simulink model "frame_inspector_test"  (R2020a)
settings: Solver=VariableStepAuto  StartTime=0.0  StopTime=(4096*6)/1e6  RelTol=1e-3
undefined symbols (not defined in the file): frame_size
libraries: hdlsllib x3, dspsrcs4 x2, dspsigops x2
settings Model: Creator=LDM  LastModifiedBy=LDM
settings OptimizationCC: BlockReduction=off  ConditionallyExecuteInputs=off  DefaultParameterBehavior=Inlined
settings DebuggingCC: AlgebraicLoopMsg=error
settings HardwareCC: ProdBitPerPointer=32  ProdBitPerSizeT=32  ProdBitPerPtrDiffT=32  ProdLargestAtomicFloat=None  ProdIntDivRoundTo=Undefined  ProdEndianess=Unspecified  ProdWordSize=32  ProdHWDeviceType=ASIC/FPGA->ASIC/FPGA  TargetBitPerPointer=64  TargetBitPerSizeT=64  TargetBitPerPtrDiffT=64  TargetLongLongMode=on  TargetIntDivRoundTo=Zero  TargetEndianess=LittleEndian  TargetWordSize=64  TargetHWDeviceType=Custom Processor->MATLAB Host Computer  ProdEqTarget=off

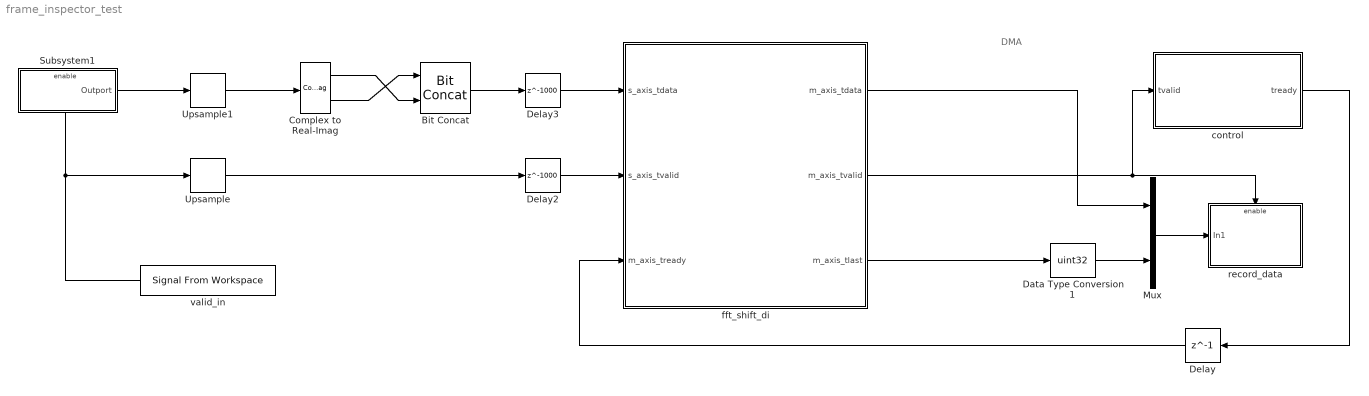
== system frame_inspector_test ==
  note: DMA
  Bit Concat : hdlsllib/Logic and Bit Operations/Bit Concat  numInputs=2
  Complex to Real-Imag : ComplexToRealImag
  Data Type Conversion1 : DataTypeConversion  OutDataTypeStr=uint32
  Delay : Delay  DelayLength=1
  Delay2 : Delay  DelayLength=1000
  Delay3 : Delay  DelayLength=1000
  Mux : Mux  Inputs=2
  Subsystem1 : Subsystem
  Upsample : dspsigops/Upsample  N=12  phase=0  RateOptions=Allow multirate processing  ic=0  mode=Unused parameter value
  Upsample1 : dspsigops/Upsample  N=12  phase=0  RateOptions=Allow multirate processing  ic=0  mode=Unused parameter value
  control : Stateflow chart  TreatAsAtomicUnit=on
  fft_shift_di : Subsystem  TreatAsAtomicUnit=on
  record_data : Subsystem
  valid_in : dspsrcs4/Signal From Workspace  X=[true(1,randi(10)) false(1,randi(10)) true(1,randi(10))]  Ts=1/1e6  nsamps=1  OutputAfterFinalValue=Cyclic repetition  ignoreOrWarnInputAndFrameLengths=off  OutputFrames=off
  wires:
  control/1(tready) -> Delay/1
  Subsystem1/1(Outport) -> Upsample1/1
  valid_in/1 -> Upsample/1, Subsystem1/Enable
  Upsample1/1 -> Complex to Real-Imag/1
  Delay/1 -> fft_shift_di/3(m_axis_tready)
  Mux/1 -> record_data/1(In1)
  fft_shift_di/1(m_axis_tdata) -> Mux/1
  Complex to Real-Imag/1 -> Bit Concat/2
  Complex to Real-Imag/2 -> Bit Concat/1
  Upsample/1 -> Delay2/1
  fft_shift_di/2(m_axis_tvalid) -> control/1(tvalid), record_data/Enable
  fft_shift_di/3(m_axis_tlast) -> Data Type Conversion1/1
  Data Type Conversion1/1 -> Mux/2
  Bit Concat/1 -> Delay3/1
  Delay2/1 -> fft_shift_di/2(s_axis_tvalid)
  Delay3/1 -> fft_shift_di/1(s_axis_tdata)

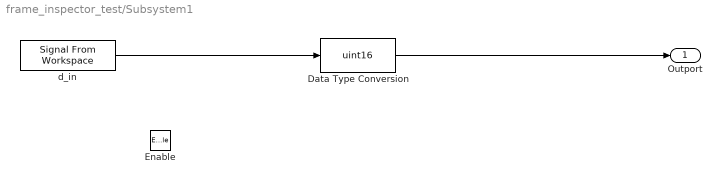
== system frame_inspector_test/Subsystem1 ==
  Enable : EnablePort
  Data Type Conversion : DataTypeConversion  OutDataTypeStr=uint16
  d_in : dspsrcs4/Signal From Workspace  X=1:frame_size  Ts=1/1e6  nsamps=1  OutputAfterFinalValue=Cyclic repetition  ignoreOrWarnInputAndFrameLengths=off  OutputFrames=off
  Outport : Outport
  wires:
  d_in/1 -> Data Type Conversion/1
  Data Type Conversion/1 -> Outport/1

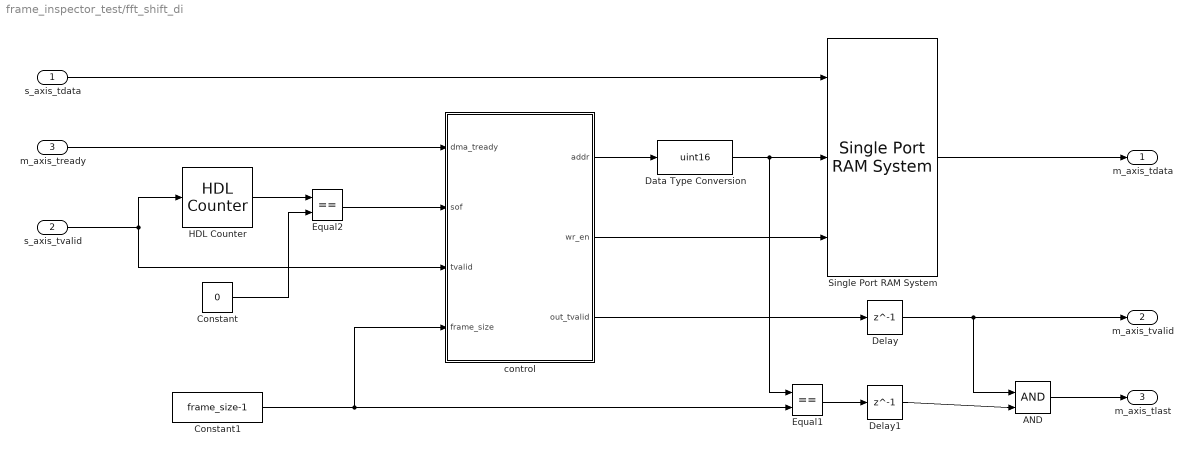
== system frame_inspector_test/fft_shift_di ==
  s_axis_tdata : Inport
  s_axis_tvalid : Inport  Port=2
  m_axis_tready : Inport  Port=3
  AND : Logic  IconShape=distinctive  AllPortsSameDT=off  OutDataTypeStr=boolean
  Constant : Constant  Value=0  OutDataTypeStr=uint16  SampleTime=-1
  Constant1 : Constant  Value=frame_size-1  OutDataTypeStr=uint16  SampleTime=-1
  Data Type Conversion : DataTypeConversion  OutDataTypeStr=uint16
  Delay : Delay  DelayLength=1
  Delay1 : Delay  DelayLength=1
  Equal1 : RelationalOperator  Operator===  OutDataTypeStr=boolean  RndMeth=Simplest
  Equal2 : RelationalOperator  Operator===  OutDataTypeStr=boolean  RndMeth=Simplest
  HDL Counter : hdlsllib/Sources/HDL Counter  CountType=Free running  CountInit=0  CountStep=1  CountMax=63  CountFromType=Initial value  CountFrom=0  CountResetPort=off  CountLoadPort=off  CountEnbPort=on  CountDirPort=off  CountDataType=Unsigned  CountWordLen=log2(frame_size)  CountFracLen=0  CountSampTime=1
  Single Port RAM System : hdlsllib/HDL RAMs/Single Port RAM System  RAMType=Single port  WriteOutputValue=New data  RAMInitialValue=0  SimulateUsing=Code generation
      settings: SourceProductBaseCode=SL
  control : Stateflow chart  TreatAsAtomicUnit=on
  m_axis_tdata : Outport
  m_axis_tvalid : Outport  Port=2
  m_axis_tlast : Outport  Port=3
  wires:
  s_axis_tvalid/1 -> control/3(tvalid), HDL Counter/1
  HDL Counter/1 -> Equal2/1
  Equal2/1 -> control/2(sof)
  Constant/1 -> Equal2/2
  s_axis_tdata/1 -> Single Port RAM System/1
  control/1(addr) -> Data Type Conversion/1
  control/2(wr_en) -> Single Port RAM System/3
  m_axis_tready/1 -> control/1(dma_tready)
  control/3(out_tvalid) -> Delay/1
  Single Port RAM System/1 -> m_axis_tdata/1
  Delay/1 -> m_axis_tvalid/1, AND/1
  Data Type Conversion/1 -> Equal1/1, Single Port RAM System/2
  Constant1/1 -> control/4(frame_size), Equal1/2
  Equal1/1 -> Delay1/1
  Delay1/1 -> AND/2
  AND/1 -> m_axis_tlast/1

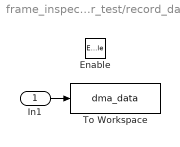
== system frame_inspector_test/record_data ==
  In1 : Inport
  Enable : EnablePort
  To Workspace : ToWorkspace  VariableName=dma_data  SampleTime=-1
      settings: Save2DSignal=2-D array (concatenate along first dimension)
  wires:
  In1/1 -> To Workspace/1

== stateflow chart frame_inspector_test/control ==
  state init
    % variables
    count = 0;
    d_count = 0;
  state start_frame
    %variables
    if tvalid == true
    d_count = d_count + 1
    end
    %outputs
    tready = true
  state wait
    % variables
    count = count + 1;
    %outputs
    tready = false
  state pause
    % variables
    count = count + 1;
    %outputs
    tready = false
  state end_frame
    %variables
    if tvalid == true
    d_count = d_count + 1
    end
    %outputs
    tready = true
  (default) -> init
  init -> wait
  wait -> start_frame : [count > randi(100)]{count = 0}
  end_frame -> wait : [d_count == frame_size]{d_count = 0}
  start_frame -> pause : [d_count == 3]
  pause -> end_frame : [count > randi(100)]{count = 0}
  data: tready output boolean; d_count local; count local; tvalid input; frame_size constant double =frame_size

== stateflow chart frame_inspector_test/fft_shift_di/control ==
  settings: executeAtInitialization=1
  state init
    % variables
    read_flag = false;
    % outputs
    addr=-1;
    wr_en = false;
    out_tvalid = false
  state write
    % variables
    if dma_tready
    read_flag = true;
    end
    % outputs
    addr=addr+1;
    wr_en = true;
    out_tvalid = false
  state idle
    % variables
    if dma_tready
    read_flag = true;
    end
    % outputs
    addr=addr;
    wr_en = false;
    out_tvalid = false
  state wait_update
    % variables
    % outputs
    addr=addr;
    wr_en = false;
    out_tvalid = false
  state wait
    % variables
    if dma_tready
    read_flag = true;
    end
    % outputs
    addr=addr;
    wr_en = false;
    out_tvalid = false
  state read
    % variables
    % outputs
    addr=addr+1;
    wr_en = false;
    out_tvalid = true
  state read_idle
    % variables
    % outputs
    addr=addr;
    wr_en = false;
    out_tvalid = false
  (default) -> init
  init -> write : [sof && tvalid]
  wait_update -> write : [sof && tvalid]
  wait -> write [order 1] : [sof && tvalid]
  write -> idle [order 3] : [~tvalid]
  idle -> write : [tvalid]
  write -> wait [order 2] : [addr==frame_size]
  write -> read [order 1] : [read_flag && addr==frame_size]{read_flag=false;addr=-1}
  read -> wait_update [order 1] : [addr==frame_size]{addr=-1}
  wait -> read [order 2] : [read_flag]{read_flag=false; addr=-1}
  read_idle -> read : [dma_tready]
  read -> read_idle [order 2] : [~dma_tready]
  data: dma_tready input boolean; sof input; addr output int16; wr_en output boolean; tvalid input; out_tvalid output; read_flag local; frame_size input
